simulink model "controller_for_carsimROS"  (R2021a)
settings: Solver=VariableStepAuto  StartTime=0.0  StopTime=15  RelTol=1e-2
values from neighbouring files (symbols this model uses):
  Fyf = zeros(1,57)    [FyfLookUpNewCar.m]    (also in Fyf_loopup_table.mat = [-9372.31873381 -9371.87234491 -9368.75632133 -9360.32413915)
  SlipAngle = -SlipAngle    [FyfLookUpNewCar.m]    (also in Fyf_loopup_table.mat = [0.153111393254 0.147643129209 0.142174865164 0.13670660112 )
  Vx = 15    [controller_setup.m]
libraries: robotlib x17, Solver_SF x1, simulink_extras x1, simulink x1
settings Model: Creator=dekunw  LastModifiedBy=chnwa
settings SolverCC: AlgebraicLoopSolver=LineSearch
settings DebuggingCC: SFMachineParentedDataDiag=warning

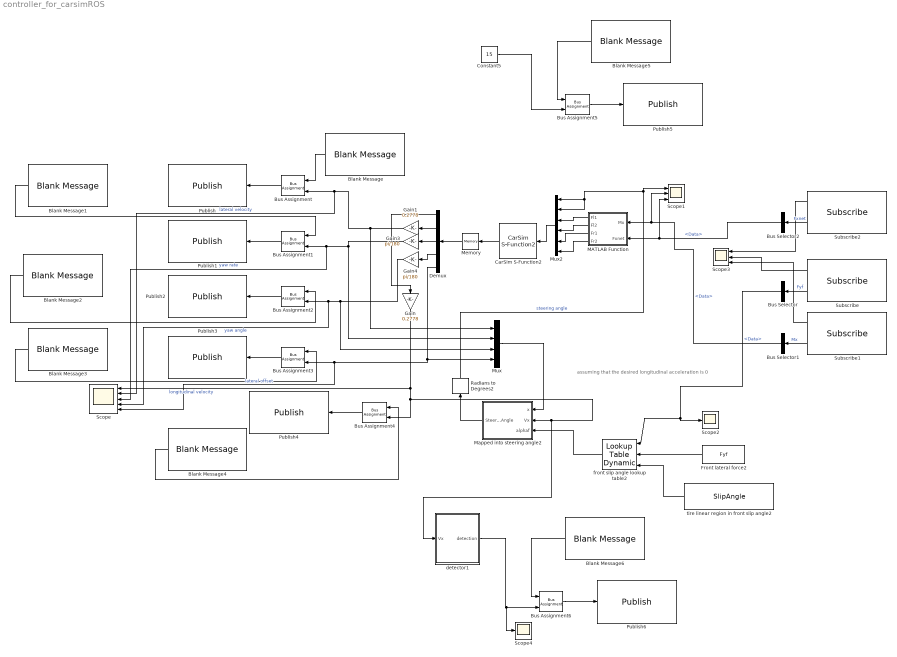
== system controller_for_carsimROS ==
  note: assuming that the desired longitudinal acceleration is 0
  Blank Message{,1..6} (7 alike) : robotlib/Blank Message  messageClass=Message  entityType=std_msgs/Float64  messageType=std_msgs/Float64  SampleTime=inf  legacyBusStruct=off
  Bus Assignment{,1..6} (7 alike) : BusAssignment  AssignedSignals=Data
  Bus Selector : BusSelector  OutputSignals=Data
  Bus Selector1 : BusSelector  OutputSignals=Data
  Bus Selector2 : BusSelector  OutputSignals=Data
  CarSim S-Function2 : Solver_SF/CarSim S-Function2  Priority=1  VehicleCode=i_i  SIMFILE=simfile.sim
      settings: AttributesFormatString=Vehicle Code: %<VehicleCode>
  Constant5 : Constant  Value=15
  Demux : Demux  Outputs=5
  Front lateral force2 : Constant  Value=Fyf
  Gain : Gain  Gain=0.2778
  Gain1 : Gain  Gain=0.2778
  Gain3 : Gain  Gain=pi/180
  Gain4 : Gain  Gain=pi/180
  MATLAB Function : MATLAB Function  TreatAsAtomicUnit=on
  Mapped into steering angle2 : MATLAB Function  TreatAsAtomicUnit=on
  Memory : Memory  InitialCondition=[54 0 0 0 0]'
  Mux : Mux
  Mux2 : Mux  Inputs=6
  Publish : robotlib/Publish  topicSource=Specify your own  topic=/states1  messageType=std_msgs/Float64  legacyBusStruct=off  messageQueueLength=1
  Publish1 : robotlib/Publish  topicSource=Specify your own  topic=/states2  messageType=std_msgs/Float64  legacyBusStruct=off  messageQueueLength=1
  Publish2 : robotlib/Publish  topicSource=Specify your own  topic=/states3  messageType=std_msgs/Float64  legacyBusStruct=off  messageQueueLength=1
  Publish3 : robotlib/Publish  topicSource=Specify your own  topic=/states4  messageType=std_msgs/Float64  legacyBusStruct=off  messageQueueLength=1
  Publish4 : robotlib/Publish  topicSource=Specify your own  topic=/Vx  messageType=std_msgs/Float64  legacyBusStruct=off  messageQueueLength=1
  Publish5 : robotlib/Publish  topicSource=Specify your own  topic=/Vset  messageType=std_msgs/Float64  legacyBusStruct=off  messageQueueLength=1
  Publish6 : robotlib/Publish  topicSource=Specify your own  topic=/detection  messageType=std_msgs/Float64  legacyBusStruct=off  messageQueueLength=1
  Radians to Degrees2 : simulink_extras/Transformations/Radians to Degrees
  Scope : Scope  NumInputPorts=5
  Scope1 : Scope  NumInputPorts=3
  Scope2 : Scope
  Scope3 : Scope  NumInputPorts=3
  Scope4 : Scope
  Subscribe : robotlib/Subscribe  topicSource=Specify your own  topic=/mv1  messageType=std_msgs/Float64  SampleTime=-1  legacyBusStruct=off  messageQueueLength=1
  Subscribe1 : robotlib/Subscribe  topicSource=Specify your own  topic=/mv2  messageType=std_msgs/Float64  SampleTime=-1  legacyBusStruct=off  messageQueueLength=1
  Subscribe2 : robotlib/Subscribe  topicSource=Specify your own  topic=/Fxnet  messageType=std_msgs/Float64  SampleTime=-1  legacyBusStruct=off  messageQueueLength=1
  detector1 : Subsystem
  front slip angle lookup table2 : simulink/Lookup Tables/Lookup Table Dynamic  LookUpMeth=Interpolation-Use End Values  OutDataType=fixdt('double')  OutScaling=[]  OutputDataTypeScalingMode=Specify via dialog  OutDataTypeStr=double  DoSatur=off
  tire linear region in front slip angle2 : Constant  Value=SlipAngle
  wires:
  Bus Selector1/1 -> Scope1/2, MATLAB Function/1(Mx)  "<Data>"
  tire linear region in front slip angle2/1 -> front slip angle lookup table2/3
  Bus Selector/1 -> Scope2/1, front slip angle lookup table2/1  "<Data>"
  Front lateral force2/1 -> front slip angle lookup table2/2
  Radians to Degrees2/1 -> Mux2/2, Mux2/1, Scope1/1  "steering angle"
  front slip angle lookup table2/1 -> Mapped into steering angle2/3(alphaf)
  Mapped into steering angle2/1(SteeringAngle) -> Radians to Degrees2/1
  Constant5/1 -> Bus Assignment5/2
  Demux/1 -> Gain/1
  Gain1/1 -> Scope/2, Bus Assignment/2, Mux/1  "lateral velocity"
  Gain3/1 -> Mux/2, Scope/3, Bus Assignment1/2  "yaw rate"
  Demux/4 -> Gain4/1
  Demux/5 -> Scope/5, Bus Assignment3/2, Mux/4  "lateral offset"
  Mux2/1 -> CarSim S-Function2/1
  CarSim S-Function2/1 -> Memory/1
  Gain/1 -> detector1/1(Vx), Mapped into steering angle2/2(Vx), Bus Assignment4/2, Scope/1  "longitudinal velocity"
  Demux/2 -> Gain1/1
  Demux/3 -> Gain3/1
  Gain4/1 -> Mux/3, Scope/4, Bus Assignment2/2  "yaw angle"
  MATLAB Function/1(Fl1) -> Mux2/3
  MATLAB Function/2(Fl2) -> Mux2/4
  MATLAB Function/3(Fr1) -> Mux2/5
  MATLAB Function/4(Fr2) -> Mux2/6
  Blank Message/1 -> Bus Assignment/1
  Bus Assignment/1 -> Publish/1
  Bus Assignment1/1 -> Publish1/1
  Bus Assignment2/1 -> Publish2/1
  Bus Assignment3/1 -> Publish3/1
  Bus Assignment4/1 -> Publish4/1
  Subscribe/1 -> Scope3/2
  Subscribe/2 -> Bus Selector/1  "Fyf"
  Subscribe1/1 -> Scope3/3
  Subscribe1/2 -> Bus Selector1/1  "Mx"
  Bus Assignment5/1 -> Publish5/1
  Subscribe2/1 -> Scope3/1
  Subscribe2/2 -> Bus Selector2/1  "Fxnet"
  Bus Selector2/1 -> Scope1/3, MATLAB Function/2(Fxnet)  "<Data>"
  Mux/1 -> Mapped into steering angle2/1(x)
  Blank Message1/1 -> Bus Assignment1/1
  Blank Message2/1 -> Bus Assignment2/1
  Blank Message3/1 -> Bus Assignment3/1
  Blank Message4/1 -> Bus Assignment4/1
  Blank Message5/1 -> Bus Assignment5/1
  Blank Message6/1 -> Bus Assignment6/1
  Bus Assignment6/1 -> Publish6/1
  detector1/1(detection) -> Scope4/1, Bus Assignment6/2
  Memory/1 -> Demux/1

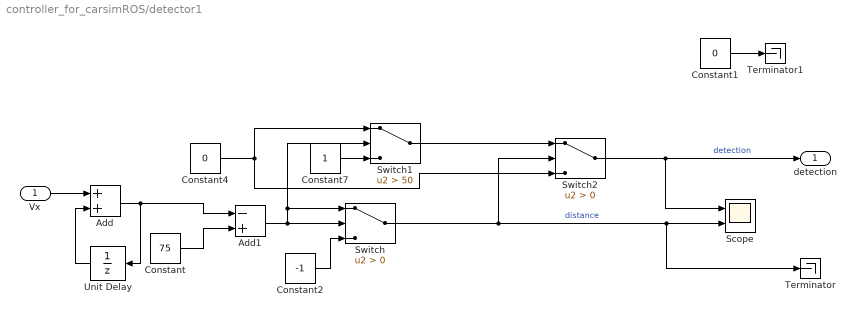
== system controller_for_carsimROS/detector1 ==
  Vx : Inport
  Add : Sum
  Add1 : Sum  Inputs=-+
  Constant : Constant  Value=75
  Constant1 : Constant  Value=0
  Constant2 : Constant  Value=-1
  Constant4 : Constant  Value=0
  Constant7 : Constant
  Scope : Scope  NumInputPorts=2
  Switch : Switch  Criteria=u2 > Threshold
  Switch1 : Switch  Criteria=u2 > Threshold  Threshold=50
  Switch2 : Switch  Criteria=u2 > Threshold
  Terminator : Terminator
  Terminator1 : Terminator
  Unit Delay : UnitDelay  SampleTime=-1  HasFrameUpgradeWarning=on
  detection : Outport
  wires:
  Constant2/1 -> Switch/3
  Constant4/1 -> Switch2/3, Switch1/1
  Vx/1 -> Add/1
  Add/1 -> Add1/1, Unit Delay/1
  Switch/1 -> Switch2/2, Terminator/1, Scope/2  "distance"
  Constant7/1 -> Switch1/3
  Add1/1 -> Switch1/2, Switch/1, Switch/2
  Switch1/1 -> Switch2/1
  Constant/1 -> Add1/2
  Switch2/1 -> detection/1, Scope/1  "detection"
  Constant1/1 -> Terminator1/1
  Unit Delay/1 -> Add/2

== matlab function controller_for_carsimROS/Mapped into steering angle2 ==
  data: x input; Vx input; alphaf input; SteeringAngle output
function SteeringAngle = fcn(x,Vx, alphaf)

lf = 1.11;  % distance from front axle to the mass center

Vy = x(1); %lateral velocity
r = x(2);  %yaw rate
SteeringAngle = Vy/Vx+lf*r/Vx-alphaf;

== matlab function controller_for_carsimROS/MATLAB Function ==
  data: Fl1 output; Mx input; Fl2 output; Fxnet input; Fr1 output; Fr2 output
function [Fl1,Fl2,Fr1,Fr2] = fcn(Mx,Fxnet)

w = 1.875; % the width of the car

Fwf = zeros(2,1);
Fwr = zeros(2,1);

if Mx > 0
    Fwf(1) = Fxnet/2+0;
    Fwf(2) = Fxnet/2-Mx/w;
    Fwr(1) = 0;
    Fwr(2) = -Mx/w;
elseif Mx < 0
    Fwf(1) = Fxnet/2+Mx/w;
    Fwf(2) = Fxnet/2+0;
    Fwr(1) = Mx/w;
    Fwr(2) = 0;
else
    Fwf(1) = Fxnet/2+0;
    Fwf(2) = Fxnet/2+0;
    Fwr(1) = 0;
    Fwr(2) = 0;
end
Fl1 = Fwf(1);
Fl2 = Fwr(1);
Fr1 = Fwf(2);
Fr2 = Fwr(2);
